simulink model "myss_p1_ej3"  (R2022b)
settings: Solver=VariableStepAuto  StartTime=0.0  StopTime=946100000.000  RelTol=1e-3
settings Model: Creator=adrub  LastModifiedBy=adrub

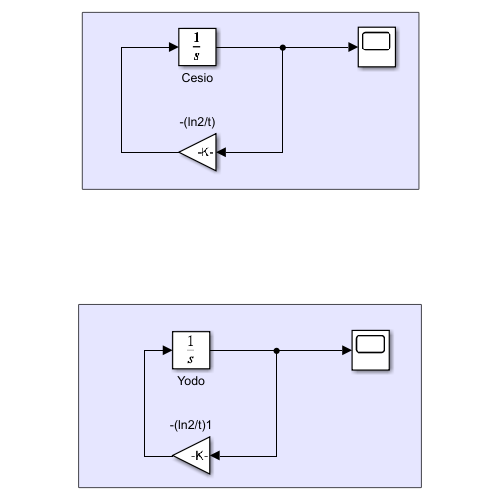
[thumbnail: Simulink's stored preview of the top-level diagram]
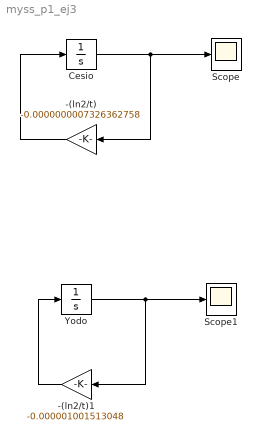
== system myss_p1_ej3 ==
  -(ln2/t) : Gain  Gain=-0.0000000007326362758
  -(ln2/t)1 : Gain  Gain=-0.000001001513048
  Cesio : Integrator  InitialCondition=1000
  Scope : Scope
  Scope1 : Scope
  Yodo : Integrator  InitialCondition=100000
  wires:
  Cesio/1 -> -(ln2/t)/1, Scope/1
  -(ln2/t)/1 -> Cesio/1
  -(ln2/t)1/1 -> Yodo/1
  Yodo/1 -> -(ln2/t)1/1, Scope1/1
